simulink model "controller_stateflow"  (R2022b)
settings: Solver=FixedStepAuto  StartTime=0.0  StopTime=inf  FixedStep=0.05  RelTol=1e-3
PreLoadFcn:
  | rosinit();
model workspace (MAT data in the model file):
  SL_ROS_VariableLengthArrays_MaxSizes.CommonInfo.ArrayTruncateAction = 'EmitWarning'
  SL_ROS_VariableLengthArrays_MaxSizes.MsgTypeMap = containers.Map
  SL_ROS_VariableLengthArrays_MaxSizes.MsgTypeMap.serialization.keys = {'gazebo_msgs/LinkStates', 'trajectory_msgs/JointTrajectory', 'trajectory_msgs/JointTrajectoryPoint'}
  SL_ROS_VariableLengthArrays_MaxSizes.MsgTypeMap.serialization.values{1}(1).PropertyName = 'Name'
  SL_ROS_VariableLengthArrays_MaxSizes.MsgTypeMap.serialization.values{1}(1).DataType = 'std_msgs/String'
  SL_ROS_VariableLengthArrays_MaxSizes.MsgTypeMap.serialization.values{1}(1).MaxLength = 100
  SL_ROS_VariableLengthArrays_MaxSizes.MsgTypeMap.serialization.values{1}(2).PropertyName = 'Pose'
  SL_ROS_VariableLengthArrays_MaxSizes.MsgTypeMap.serialization.values{1}(2).DataType = 'geometry_msgs/Pose'
  SL_ROS_VariableLengthArrays_MaxSizes.MsgTypeMap.serialization.values{1}(2).MaxLength = 100
  SL_ROS_VariableLengthArrays_MaxSizes.MsgTypeMap.serialization.values{1}(3).PropertyName = 'Twist'
  SL_ROS_VariableLengthArrays_MaxSizes.MsgTypeMap.serialization.values{1}(3).DataType = 'geometry_msgs/Twist'
  SL_ROS_VariableLengthArrays_MaxSizes.MsgTypeMap.serialization.values{1}(3).MaxLength = 100
  SL_ROS_VariableLengthArrays_MaxSizes.MsgTypeMap.serialization.values{2}(1).PropertyName = 'JointNames'
  SL_ROS_VariableLengthArrays_MaxSizes.MsgTypeMap.serialization.values{2}(1).DataType = 'std_msgs/String'
  SL_ROS_VariableLengthArrays_MaxSizes.MsgTypeMap.serialization.values{2}(1).MaxLength = 16
  SL_ROS_VariableLengthArrays_MaxSizes.MsgTypeMap.serialization.values{2}(2).PropertyName = 'Points'
  SL_ROS_VariableLengthArrays_MaxSizes.MsgTypeMap.serialization.values{2}(2).DataType = 'trajectory_msgs/JointTrajectoryPoint'
  SL_ROS_VariableLengthArrays_MaxSizes.MsgTypeMap.serialization.values{2}(2).MaxLength = 5
  SL_ROS_VariableLengthArrays_MaxSizes.MsgTypeMap.serialization.values{3}(1).PropertyName = 'Accelerations'
  SL_ROS_VariableLengthArrays_MaxSizes.MsgTypeMap.serialization.values{3}(1).DataType = 'double'
  SL_ROS_VariableLengthArrays_MaxSizes.MsgTypeMap.serialization.values{3}(1).MaxLength = 128
  SL_ROS_VariableLengthArrays_MaxSizes.MsgTypeMap.serialization.values{3}(2).PropertyName = 'Effort'
  SL_ROS_VariableLengthArrays_MaxSizes.MsgTypeMap.serialization.values{3}(2).DataType = 'double'
  SL_ROS_VariableLengthArrays_MaxSizes.MsgTypeMap.serialization.values{3}(2).MaxLength = 128
  SL_ROS_VariableLengthArrays_MaxSizes.MsgTypeMap.serialization.values{3}(3).PropertyName = 'Positions'
  SL_ROS_VariableLengthArrays_MaxSizes.MsgTypeMap.serialization.values{3}(3).DataType = 'double'
  SL_ROS_VariableLengthArrays_MaxSizes.MsgTypeMap.serialization.values{3}(3).MaxLength = 7
  SL_ROS_VariableLengthArrays_MaxSizes.MsgTypeMap.serialization.values{3}(4).PropertyName = 'Velocities'
  SL_ROS_VariableLengthArrays_MaxSizes.MsgTypeMap.serialization.values{3}(4).DataType = 'double'
  SL_ROS_VariableLengthArrays_MaxSizes.MsgTypeMap.serialization.values{3}(4).MaxLength = 128
  SL_ROS_VariableLengthArrays_MaxSizes.MsgTypeMap.serialization.uniformity = 0
  SL_ROS_VariableLengthArrays_MaxSizes.MsgTypeMap.serialization.keyType = 'char'
  SL_ROS_VariableLengthArrays_MaxSizes.MsgTypeMap.serialization.valueType = 'any'
  pitch = -10
  restart = 0
undefined symbols (not defined in the file): StartTime
libraries: robotmaniplib x62, robotlib x17, robotcorelib x4, robotgazebolib x1
(part 1 of 4)
settings Model: Creator=marco  LastModifiedBy=marco
settings OptimizationCC: EnhancedBackFolding=on  PassReuseOutputArgsAs=Individual arguments  ZeroExternalMemoryAtStartup=off  ZeroInternalMemoryAtStartup=off  MaxStackSize=64  OptimizeBlockOrder=speed  DifferentSizesBufferReuse=on  OptimizationCustomize=off  EfficientTunableParamExpr=on
settings DebuggingCC: ParameterTunabilityLossMsg=error
settings HardwareCC: ProdBitPerPointer=32  ProdBitPerSizeT=32  ProdBitPerPtrDiffT=32  ProdLargestAtomicFloat=None  ProdIntDivRoundTo=Undefined  ProdEndianess=Unspecified  ProdWordSize=32  ProdHWDeviceType=Generic->Unspecified (assume 32-bit Generic)
settings SFSimCC: MATLABDynamicMemAlloc=off
settings RTWCC: Description=Embedded Coder  SystemTargetFile=ert.tlc  HardwareBoard=Robot Operating System (ROS)  TLCOptions="-aInlineSetEventsForThisBaseRateFcn=TLC_FALSE -aSuppressMultiTaskScheduler=TLC_FALSE  -aRateBasedStepFcn=0"  TemplateMakefile=ert_default_tmf  Toolchain=Catkin  TargetLang=C++
settings CodeAppCC: ForceParamTrailComments=on  IgnoreCustomStorageClasses=off  OperatorAnnotations=on  SimulinkDataObjDesc=on  SFDataObjDesc=on  InsertBlockDesc=on

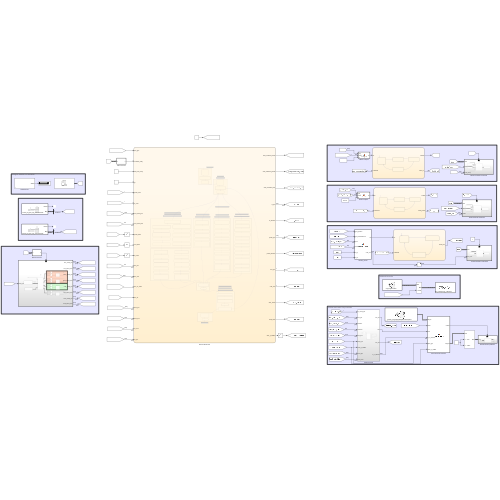
[thumbnail: Simulink's stored preview of the top-level diagram]
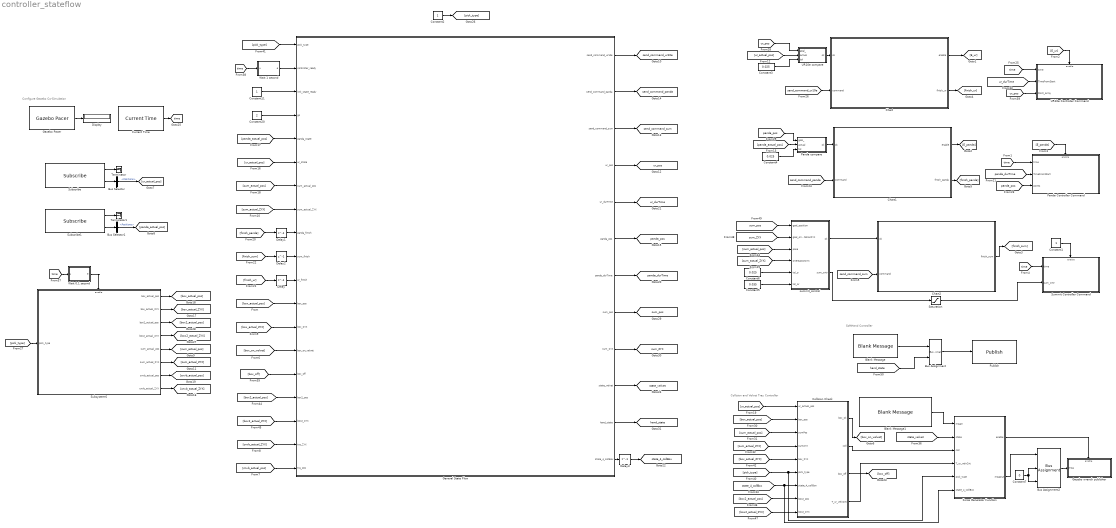
== system controller_stateflow ==
  note: Collision and Velvet Tray Controller
  note: SoftHand Controller
  note: Configure Gazebo Co-Simulation
  Blank Message : robotlib/Blank Message  messageClass=Message  entityType=std_msgs/Float64  messageType=std_msgs/Float64  SampleTime=inf  legacyBusStruct=off
      settings: LibrarySourceBlock=roslib/ROS/Blank Message
  Blank Message1 : robotlib/Blank Message  messageClass=Service Request  entityType=gazebo_msgs/ApplyBodyWrench  messageType=gazebo_msgs/ApplyBodyWrenchRequest  SampleTime=-1  legacyBusStruct=off
      settings: LibrarySourceBlock=roslib/ROS/Blank Message
  Bus Assignment : BusAssignment  AssignedSignals=Data
  Bus Assignment2 : BusAssignment  AssignedSignals=StartTime.Sec,StartTime.Nsec
  Bus Selector : BusSelector  OutputSignals=Actual.Positions
  Bus Selector1 : BusSelector  OutputSignals=Actual.Positions
  Chart : Stateflow chart  TreatAsAtomicUnit=on
  Chart1 : Stateflow chart  TreatAsAtomicUnit=on
  Chart2 : Stateflow chart  TreatAsAtomicUnit=on
  Collision Check : Subsystem
  Constant1 : Constant
  Constant11 : Constant
  Constant2 : Constant
  Constant20 : Constant  Value=2
  Constant3 : Constant  Value=0.025
  Constant4 : Constant  Value=0.025
  Constant5 : Constant  Value=0.035
  Constant6 : Constant  Value=0.025
  Constant7 : Constant  Value=0
  Current Time : robotlib/Current Time  OutputFormat=bus  SampleTime=-1  ModelName=controller_stateflow
      settings: LibrarySourceBlock=roslib/ROS/Current Time
  Delay{,1..3} (4 alike) : Delay  DelayLength=1  InitialCondition=0
  Display : Display
  Force Generator Function : MATLAB Function  TreatAsAtomicUnit=on
  Gazebo Pacer : robotgazebolib/Gazebo Pacer  ResetBehavior=Reset Gazebo simulation time  SampleTime=0.05
  Gazebo wrench publisher : Subsystem
  General State Flow : Stateflow chart  TreatAsAtomicUnit=on
  Panda Controller Command : Subsystem
  Panda compare : MATLAB Function  TreatAsAtomicUnit=on
  Publish : robotlib/Publish  topicSource=Select from ROS network  topic=/right_hand_v1s/synergy_command  messageType=std_msgs/Float64  legacyBusStruct=off  messageQueueLength=1
      settings: LibrarySourceBlock=roslib/ROS/Publish
  Saturation : Saturate  UpperLimit=0.3  LowerLimit=-0.3
  Subscribe : robotlib/Subscribe  topicSource=Select from ROS network  topic=/ur10e_eff_joint_traj_controller/state  messageType=control_msgs/JointTrajectoryControllerState  SampleTime=-1  legacyBusStruct=off  messageQueueLength=1
      settings: LibrarySourceBlock=roslib/ROS/Subscribe
  Subscribe1 : robotlib/Subscribe  topicSource=Select from ROS network  topic=/panda_eff_joint_traj_controller/state  messageType=control_msgs/JointTrajectoryControllerState  SampleTime=-1  legacyBusStruct=off  messageQueueLength=1
      settings: LibrarySourceBlock=roslib/ROS/Subscribe
  Subsystem6 : Subsystem
  Summit Controller Command : Subsystem
  Terminator : Terminator
  Terminator1 : Terminator
  UR10e Controller Command : Subsystem
  UR10e compare : MATLAB Function  TreatAsAtomicUnit=on
  Wait 0,1 second : MATLAB Function  TreatAsAtomicUnit=on
  Wait 1 second : MATLAB Function  TreatAsAtomicUnit=on
  summit_control : MATLAB Function  TreatAsAtomicUnit=on
  tag scope: hand_state=global, panda_durTime=global, panda_pos=global, send_command_panda=global, send_command_sum=global, send_command_ur10e=global, state_4_collBox=global, state_velvet=global, sum_ZYX=global, sum_pos=global, time=global, ur_durTime=global, ur_pos=global
  wires:
  [time] -> Panda Controller Command/1(time)
  [E_ur] -> UR10e Controller Command/Enable
  Chart/1(enable) -> [E_ur]
  Subscribe/2 -> Bus Selector/1
  Constant3/1 -> UR10e compare/3(tol)
  UR10e compare/1(ok) -> Chart/1(ok)
  Panda compare/1(ok) -> Chart1/1(ok)
  Constant4/1 -> Panda compare/3(tol)
  Subscribe1/2 -> Bus Selector1/1
  [panda_pos] -> Panda Controller Command/3(points)
  Constant6/1 -> summit_control/5(tol_p)
  summit_control/1(ok) -> Chart2/1(ok)
  summit_control/2(sum_cntr) -> Saturation/1
  Constant1/1 -> Summit Controller Command/Enable
  Chart/2(finish_ur) -> [finish_ur]
  Saturation/1 -> Summit Controller Command/2(sum_cntr)
  Wait 0,1 second/1(e) -> Subsystem6/Enable
  Constant11/1 -> General State Flow/3(link_state_ready)
  Bus Selector/1 -> [ur_actual_pos]  "<Positions>"
  Bus Selector1/1 -> [panda_actual_pos]  "<Positions>"
  [ur_actual_pos] -> UR10e compare/2(actual)
  [sum_actual_ZYX] -> summit_control/4(orientationZYX)
  [panda_actual_pos] -> Panda compare/2(actual)
  [panda_actual_pos] -> General State Flow/5(panda_state)
  [ur_actual_pos] -> General State Flow/6(ur_state)
  [finish_sum] -> Delay2/1
  [finish_ur] -> Delay/1
  Delay/1 -> General State Flow/11(ur_finish)
  Constant20/1 -> General State Flow/4(go)
  [time] -> UR10e Controller Command/1(time)
  General State Flow/1(send_command_ur10e) -> [send_command_ur10e]
  [send_command_ur10e] -> Chart/2(command)
  [ur_pos] -> UR10e compare/1(goal_)
  General State Flow/3(send_command_sum) -> [send_command_sum]
  General State Flow/2(send_command_panda) -> [send_command_panda]
  General State Flow/4(ur_pos) -> [ur_pos]
  General State Flow/6(panda_pos) -> [panda_pos]
  [send_command_panda] -> Chart1/2(command)
  [panda_pos] -> Panda compare/1(goal_)
  [finish_panda] -> Delay1/1
  Delay1/1 -> General State Flow/9(panda_finish)
  [time] -> Summit Controller Command/1(time)
  [send_command_sum] -> Chart2/2(command)
  Chart2/1(finish_sum) -> [finish_sum]
  Delay2/1 -> General State Flow/10(sum_finish)
  [box_actual_ZYX] -> General State Flow/13(box_ZYX)
  [box_actual_pos] -> General State Flow/12(box_pos)
  [sum_actual_pos] -> summit_control/3(pose)
  [sum_actual_ZYX] -> General State Flow/8(sum_actual_ZYX)
  [sum_actual_pos] -> General State Flow/7(sum_actual_pos)
  [box_on_velvet] -> General State Flow/14(box_on_velvet)
  Bus Assignment/1 -> Publish/1
  Blank Message/1 -> Bus Assignment/1
  [cnvb_actual_pos] -> General State Flow/19(tra_pos)
  [cnvb_actual_ZYX] -> General State Flow/18(tra_ZYX)
  [E_panda] -> Panda Controller Command/Enable
  [panda_durTime] -> Panda Controller Command/2(TimeFromStart)
  General State Flow/5(ur_durTime) -> [ur_durTime]
  [ur_durTime] -> UR10e Controller Command/2(TimeFromStart)
  General State Flow/7(panda_durTime) -> [panda_durTime]
  Force Generator Function/1(enable) -> Gazebo wrench publisher/Enable
  Blank Message1/1 -> Force Generator Function/1(msgIn)
  Bus Assignment2/1 -> Gazebo wrench publisher/1(msg)
  Constant7/1 -> Bus Assignment2/3, Bus Assignment2/2
  Force Generator Function/2(msgOut) -> Bus Assignment2/1
  [box_off] -> General State Flow/15(box_off)
  General State Flow/10(state_velvet) -> [state_velvet]
  [ur_actual_pos] -> Collision Check/1(ur_actual_pos)
  [box_actual_pos] -> Collision Check/2(box_pos)
  [sum_actual_pos] -> Collision Check/3(sumPos)
  [sum_actual_ZYX] -> Collision Check/4(sumZYX)
  Collision Check/1(box_ok) -> [box_on_velvet]
  Collision Check/2(coll) -> Force Generator Function/3(coll)
  Collision Check/3(box_off) -> [box_off]
  Collision Check/4(T_ur_velvCnt) -> Force Generator Function/4(T_ur_velvCnt)
  Gazebo Pacer/1 -> Display/1
  Subsystem6/5(sum_actual_pos) -> [sum_actual_pos]
  Subsystem6/6(sum_actual_ZYX) -> [sum_actual_ZYX]
  Subsystem6/7(cnvb_actual_pos) -> [cnvb_actual_pos]
  Subsystem6/8(cnvb_actual_ZYX) -> [cnvb_actual_ZYX]
  [time] -> Wait 0,1 second/1(u)
  Current Time/1 -> [time]
  [time] -> Wait 1 second/1(u)
  Wait 1 second/1(e) -> General State Flow/2(controller_ready)
  [ur_pos] -> UR10e Controller Command/3(Point_array)
  Constant2/1 -> [pick_type]
  Subsystem6/1(box_actual_pos) -> [box_actual_pos]
  Subsystem6/2(box_actual_ZYX) -> [box_actual_ZYX]
  [pick_type] -> Subsystem6/1(pick_type)
  [pick_type] -> Collision Check/6(pick_type), Force Generator Function/5(pick_type)
  [pick_type] -> General State Flow/1(pick_type)
  [box_actual_ZYX] -> Collision Check/5(box_ZYX)
  [state_velvet] -> Force Generator Function/2(state)
  Subsystem6/3(box2_actual_pos) -> [box2_actual_pos]
  Subsystem6/4(box2_actual_ZYX) -> [box2_actual_ZYX]
  [box2_actual_ZYX] -> General State Flow/17(box2_ZYX)
  [box2_actual_pos] -> General State Flow/16(box2_pos)
  [box2_actual_pos] -> Collision Check/8(box2_pos)
  [box2_actual_ZYX] -> Collision Check/9(box2_ZYX)
  General State Flow/12(state_4_collBox) -> Delay3/1
  Subscribe/1 -> Terminator/1
  Subscribe1/1 -> Terminator1/1
  General State Flow/9(sum_ZYX) -> [sum_ZYX]
  [sum_ZYX] -> summit_control/2(goal_orientationZYX)
  General State Flow/8(sum_pos) -> [sum_pos]
  [sum_pos] -> summit_control/1(goal_position)
  Constant5/1 -> summit_control/6(tol_or)
  General State Flow/11(hand_state) -> [hand_state]
  [hand_state] -> Bus Assignment/2
  Chart1/2(finish_panda) -> [finish_panda]
  Chart1/1(enable) -> [E_panda]
  Delay3/1 -> [state_4_collBox]
  [state_4_collBox] -> Collision Check/7(state_4_collBox), Force Generator Function/6(state_4_collBox)

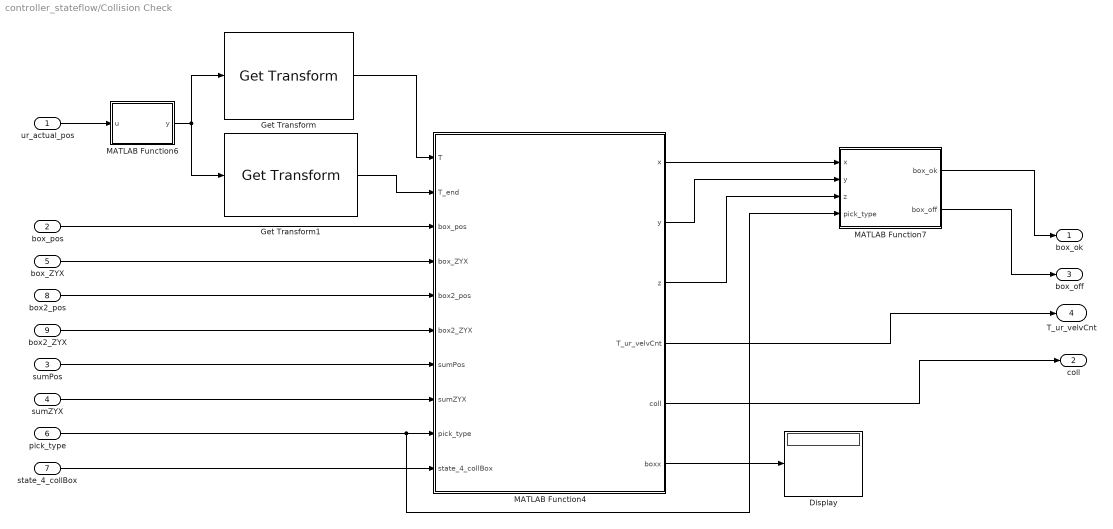
== system controller_stateflow/Collision Check ==
  ur_actual_pos : Inport
  box_pos : Inport  Port=2
  sumPos : Inport  Port=3
  sumZYX : Inport  Port=4
  box_ZYX : Inport  Port=5  OutDataTypeStr=double  PortDimensions=[3,1]
  pick_type : Inport  Port=6
  state_4_collBox : Inport  Port=7
  box2_pos : Inport  Port=8
  box2_ZYX : Inport  Port=9  OutDataTypeStr=double  PortDimensions=[3,1]
  Display : Display
  Get Transform : robotmaniplib/Get Transform  RigidBodyTree=ur10e  SourceBody=ee_link  TargetBody=world  SimulateUsing=Interpreted execution
  Get Transform1 : robotmaniplib/Get Transform  RigidBodyTree=ur10e  SourceBody=velvet_link_end  TargetBody=world  SimulateUsing=Interpreted execution
  MATLAB Function4 : MATLAB Function  TreatAsAtomicUnit=on
  MATLAB Function6 : MATLAB Function  TreatAsAtomicUnit=on
  MATLAB Function7 : MATLAB Function  TreatAsAtomicUnit=on
  box_ok : Outport
  coll : Outport  Port=2
  box_off : Outport  Port=3
  T_ur_velvCnt : Outport  Port=4
  wires:
  MATLAB Function7/1(box_ok) -> box_ok/1
  Get Transform/1 -> MATLAB Function4/1(T)
  MATLAB Function4/1(x) -> MATLAB Function7/1(x)
  MATLAB Function7/2(box_off) -> box_off/1
  MATLAB Function4/3(z) -> MATLAB Function7/3(z)
  MATLAB Function4/2(y) -> MATLAB Function7/2(y)
  MATLAB Function4/5(coll) -> coll/1
  box_pos/1 -> MATLAB Function4/3(box_pos)
  ur_actual_pos/1 -> MATLAB Function6/1(u)
  sumPos/1 -> MATLAB Function4/7(sumPos)
  MATLAB Function4/4(T_ur_velvCnt) -> T_ur_velvCnt/1
  sumZYX/1 -> MATLAB Function4/8(sumZYX)
  MATLAB Function4/6(boxx) -> Display/1
  pick_type/1 -> MATLAB Function7/4(pick_type), MATLAB Function4/9(pick_type)
  MATLAB Function6/1(y) -> Get Transform/1, Get Transform1/1
  box_ZYX/1 -> MATLAB Function4/4(box_ZYX)
  Get Transform1/1 -> MATLAB Function4/2(T_end)
  box2_ZYX/1 -> MATLAB Function4/6(box2_ZYX)
  box2_pos/1 -> MATLAB Function4/5(box2_pos)
  state_4_collBox/1 -> MATLAB Function4/10(state_4_collBox)

== system controller_stateflow/Gazebo wrench publisher ==
  msg : Inport
  Enable : EnablePort
  Call Service : robotlib/Call Service  topicSource=Select from ROS network  service=/gazebo/apply_body_wrench  serviceType=gazebo_msgs/ApplyBodyWrench  connectionTimeout=5  keepPersistent=off  ShowErrorCodeOutput=on  legacyBusStruct=off
      settings: LibrarySourceBlock=roslib/ROS/Call Service
  Terminator : Terminator
  Terminator1 : Terminator
  wires:
  Call Service/1 -> Terminator/1
  Call Service/2 -> Terminator1/1
  msg/1 -> Call Service/1

== system controller_stateflow/General State Flow/THE_END ==
  go : Inport
  Action Port : ActionPort
      settings: CopyFcn=Stateflow.SLINSF.SimulinkMan.removeBlockPreDeleteFcn  PreDeleteFcn=Stateflow.SLINSF.SimulinkMan.unsafePredeleteFcn
  Stop Simulation : Stop
  wires:
  go/1 -> Stop Simulation/1

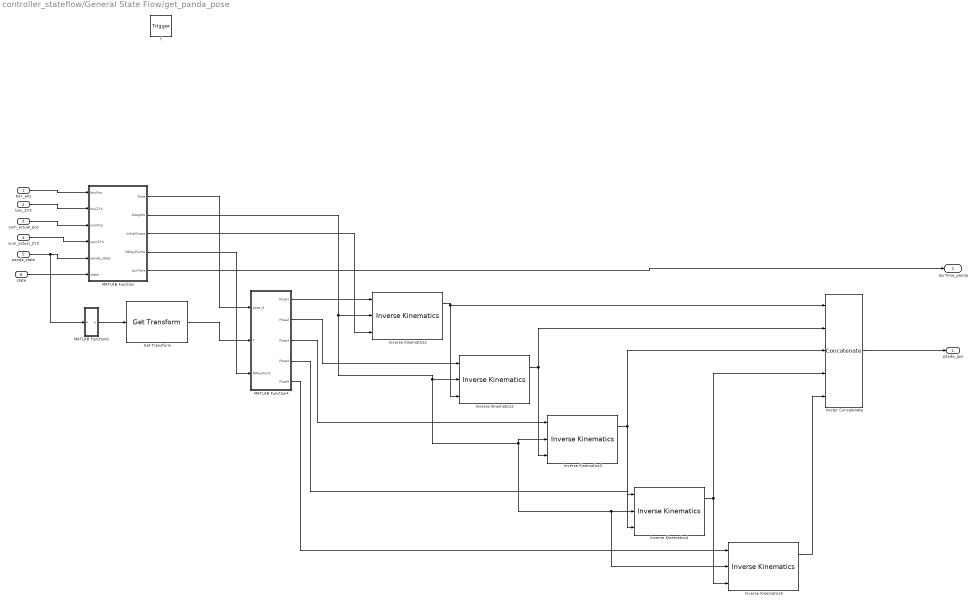
== system controller_stateflow/General State Flow/get_panda_pose ==
  box_pos : Inport  OutDataTypeStr=double  PortDimensions=[3,1]
  box_ZYX : Inport  Port=2  OutDataTypeStr=double  PortDimensions=[3,1]
  sum_actual_pos : Inport  Port=3  OutDataTypeStr=double  PortDimensions=[3,1]
  sum_actual_ZYX : Inport  Port=4  OutDataTypeStr=double  PortDimensions=[3,1]
  panda_state : Inport  Port=5  OutDataTypeStr=double  PortDimensions=[7,1]
  state : Inport  Port=6  OutDataTypeStr=double  PortDimensions=1
  f : TriggerPort  TriggerType=function-call  VariantControl=(inherit)
      settings: CopyFcn=Stateflow.SLINSF.SimulinkMan.removeBlockPreDeleteFcn  PreDeleteFcn=Stateflow.SLINSF.SimulinkMan.unsafePredeleteFcn
  Get Transform : robotmaniplib/Get Transform  RigidBodyTree=franka  SourceBody=hand_link_end  TargetBody=panda_link0  SimulateUsing=Interpreted execution
  Inverse Kinematics{1..5} (5 alike) : robotmaniplib/Inverse Kinematics  RigidBodyTree=franka  EndEffector=hand_link_end  ShowInfo=on  SolverName=BFGS Gradient Projection  EnforceJointLimits=on  MaxIterations=1500  MaxTime=10  GradientTolerance=1e-7  SolutionTolerance=1e-6  StepTolerance=1e-14  ErrorChangeTolerance=1e-12  UseErrorDamping=on  DampingBias=0.0025  SimulateUsing=Interpreted execution
  MATLAB Function : MATLAB Function  TreatAsAtomicUnit=on
  MATLAB Function4 : MATLAB Function  TreatAsAtomicUnit=on
  MATLAB Function6 : MATLAB Function  TreatAsAtomicUnit=on
  Vector Concatenate : Concatenate  NumInputs=5  Mode=Multidimensional array  ConcatenateDimension=2
  panda_pos : Outport
  durTime_panda : Outport  Port=2
  wires:
  panda_state/1 -> MATLAB Function6/1(u), MATLAB Function/5(panda_state)
  box_pos/1 -> MATLAB Function/1(boxPos)
  box_ZYX/1 -> MATLAB Function/2(boxZYX)
  sum_actual_pos/1 -> MATLAB Function/3(sumPos)
  sum_actual_ZYX/1 -> MATLAB Function/4(sumZYX)
  state/1 -> MATLAB Function/6(state)
  MATLAB Function/5(durTime) -> durTime_panda/1
  MATLAB Function/4(NWayPoints) -> MATLAB Function4/3(NWayPoint)
  Inverse Kinematics3/1 -> Inverse Kinematics4/3, Vector Concatenate/3
  MATLAB Function6/1(y) -> Get Transform/1
  Vector Concatenate/1 -> panda_pos/1
  MATLAB Function4/1(Pose1) -> Inverse Kinematics1/1
  MATLAB Function4/2(Pose2) -> Inverse Kinematics2/1
  MATLAB Function/3(initialGuess) -> Inverse Kinematics1/3
  MATLAB Function/2(Weights) -> Inverse Kinematics2/2, Inverse Kinematics3/2, Inverse Kinematics5/2, Inverse Kinematics4/2, Inverse Kinematics1/2
  MATLAB Function/1(Pose) -> MATLAB Function4/1(pose_d)
  MATLAB Function4/3(Pose3) -> Inverse Kinematics3/1
  Inverse Kinematics1/1 -> Inverse Kinematics2/3, Vector Concatenate/1
  Get Transform/1 -> MATLAB Function4/2(T)
  Inverse Kinematics2/1 -> Inverse Kinematics3/3, Vector Concatenate/2
  Inverse Kinematics4/1 -> Inverse Kinematics5/3, Vector Concatenate/4
  Inverse Kinematics5/1 -> Vector Concatenate/5
  MATLAB Function4/4(Pose4) -> Inverse Kinematics4/1
  MATLAB Function4/5(Pose5) -> Inverse Kinematics5/1

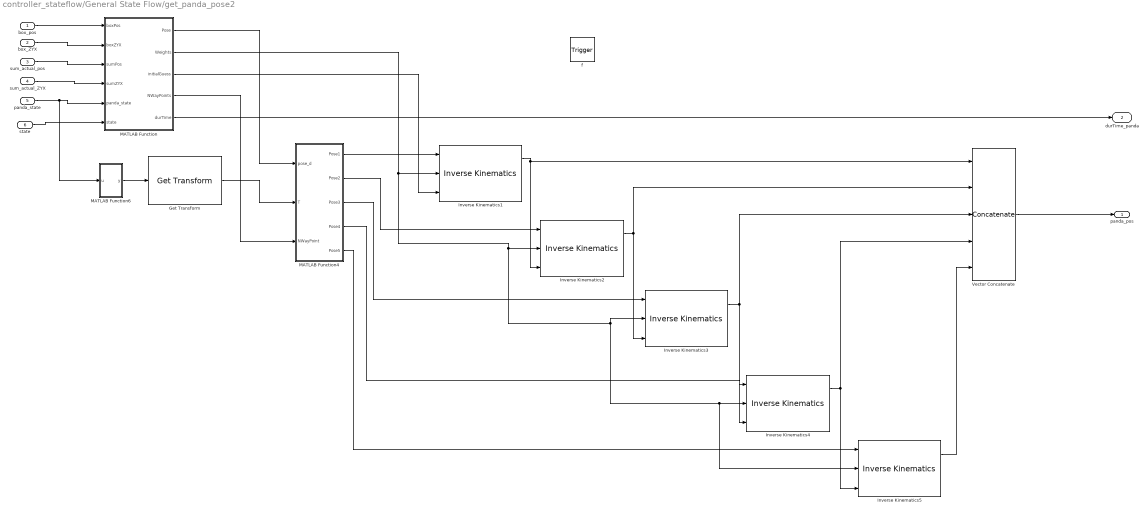
== system controller_stateflow/General State Flow/get_panda_pose2 ==
  box_pos : Inport  OutDataTypeStr=double  PortDimensions=[3,1]
  box_ZYX : Inport  Port=2  OutDataTypeStr=double  PortDimensions=[3,1]
  sum_actual_pos : Inport  Port=3  OutDataTypeStr=double  PortDimensions=[3,1]
  sum_actual_ZYX : Inport  Port=4  OutDataTypeStr=double  PortDimensions=[3,1]
  panda_state : Inport  Port=5  OutDataTypeStr=double  PortDimensions=[7,1]
  state : Inport  Port=6  OutDataTypeStr=double  PortDimensions=1
  f : TriggerPort  TriggerType=function-call  VariantControl=(inherit)
      settings: CopyFcn=Stateflow.SLINSF.SimulinkMan.removeBlockPreDeleteFcn  PreDeleteFcn=Stateflow.SLINSF.SimulinkMan.unsafePredeleteFcn
  Get Transform : robotmaniplib/Get Transform  RigidBodyTree=franka  SourceBody=hand_link_end  TargetBody=panda_link0  SimulateUsing=Interpreted execution
  Inverse Kinematics{1..5} (5 alike) : robotmaniplib/Inverse Kinematics  RigidBodyTree=franka  EndEffector=hand_link_end  ShowInfo=on  SolverName=BFGS Gradient Projection  EnforceJointLimits=on  MaxIterations=1500  MaxTime=10  GradientTolerance=1e-7  SolutionTolerance=1e-6  StepTolerance=1e-14  ErrorChangeTolerance=1e-12  UseErrorDamping=on  DampingBias=0.0025  SimulateUsing=Interpreted execution
  MATLAB Function : MATLAB Function  TreatAsAtomicUnit=on
  MATLAB Function4 : MATLAB Function  TreatAsAtomicUnit=on
  MATLAB Function6 : MATLAB Function  TreatAsAtomicUnit=on
  Vector Concatenate : Concatenate  NumInputs=5  Mode=Multidimensional array  ConcatenateDimension=2
  panda_pos : Outport
  durTime_panda : Outport  Port=2
  wires:
  panda_state/1 -> MATLAB Function6/1(u), MATLAB Function/5(panda_state)
  box_pos/1 -> MATLAB Function/1(boxPos)
  box_ZYX/1 -> MATLAB Function/2(boxZYX)
  sum_actual_pos/1 -> MATLAB Function/3(sumPos)
  sum_actual_ZYX/1 -> MATLAB Function/4(sumZYX)
  state/1 -> MATLAB Function/6(state)
  MATLAB Function/5(durTime) -> durTime_panda/1
  MATLAB Function/4(NWayPoints) -> MATLAB Function4/3(NWayPoint)
  Inverse Kinematics3/1 -> Inverse Kinematics4/3, Vector Concatenate/3
  MATLAB Function6/1(y) -> Get Transform/1
  Vector Concatenate/1 -> panda_pos/1
  MATLAB Function4/1(Pose1) -> Inverse Kinematics1/1
  MATLAB Function4/2(Pose2) -> Inverse Kinematics2/1
  MATLAB Function/3(initialGuess) -> Inverse Kinematics1/3
  MATLAB Function/2(Weights) -> Inverse Kinematics2/2, Inverse Kinematics3/2, Inverse Kinematics5/2, Inverse Kinematics4/2, Inverse Kinematics1/2
  MATLAB Function/1(Pose) -> MATLAB Function4/1(pose_d)
  MATLAB Function4/3(Pose3) -> Inverse Kinematics3/1
  Inverse Kinematics1/1 -> Inverse Kinematics2/3, Vector Concatenate/1
  Get Transform/1 -> MATLAB Function4/2(T)
  Inverse Kinematics2/1 -> Inverse Kinematics3/3, Vector Concatenate/2
  Inverse Kinematics4/1 -> Inverse Kinematics5/3, Vector Concatenate/4
  Inverse Kinematics5/1 -> Vector Concatenate/5
  MATLAB Function4/4(Pose4) -> Inverse Kinematics4/1
  MATLAB Function4/5(Pose5) -> Inverse Kinematics5/1

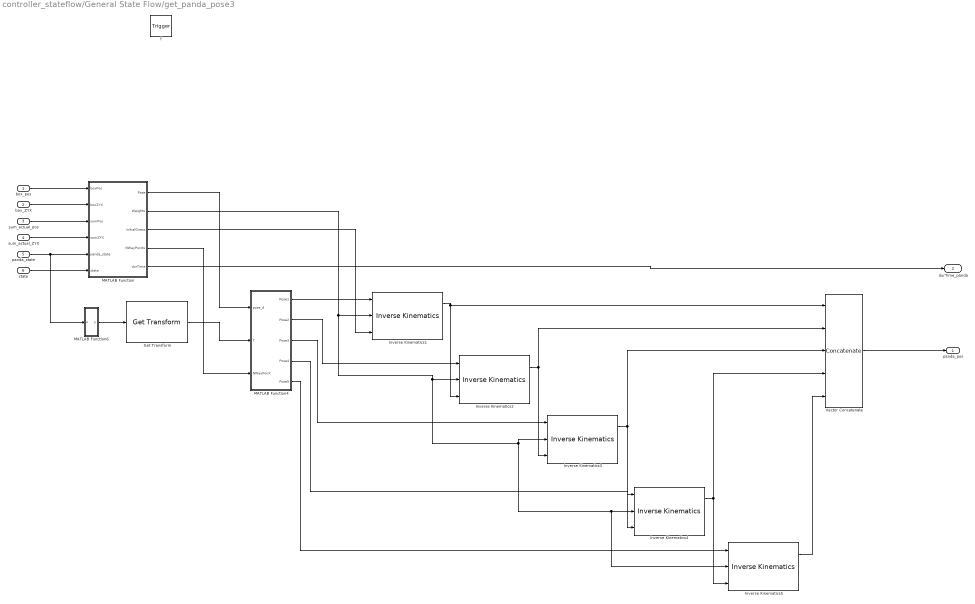
== system controller_stateflow/General State Flow/get_panda_pose3 ==
  box_pos : Inport  OutDataTypeStr=double  PortDimensions=[3,1]
  box_ZYX : Inport  Port=2  OutDataTypeStr=double  PortDimensions=[3,1]
  sum_actual_pos : Inport  Port=3  OutDataTypeStr=double  PortDimensions=[3,1]
  sum_actual_ZYX : Inport  Port=4  OutDataTypeStr=double  PortDimensions=[3,1]
  panda_state : Inport  Port=5  OutDataTypeStr=double  PortDimensions=[7,1]
  state : Inport  Port=6  OutDataTypeStr=double  PortDimensions=1
  f : TriggerPort  TriggerType=function-call  VariantControl=(inherit)
      settings: CopyFcn=Stateflow.SLINSF.SimulinkMan.removeBlockPreDeleteFcn  PreDeleteFcn=Stateflow.SLINSF.SimulinkMan.unsafePredeleteFcn
  Get Transform : robotmaniplib/Get Transform  RigidBodyTree=franka  SourceBody=hand_link_end  TargetBody=panda_link0  SimulateUsing=Interpreted execution
  Inverse Kinematics{1..5} (5 alike) : robotmaniplib/Inverse Kinematics  RigidBodyTree=franka  EndEffector=hand_link_end  ShowInfo=on  SolverName=BFGS Gradient Projection  EnforceJointLimits=on  MaxIterations=1500  MaxTime=10  GradientTolerance=1e-7  SolutionTolerance=1e-6  StepTolerance=1e-14  ErrorChangeTolerance=1e-12  UseErrorDamping=on  DampingBias=0.0025  SimulateUsing=Interpreted execution
  MATLAB Function : MATLAB Function  TreatAsAtomicUnit=on
  MATLAB Function4 : MATLAB Function  TreatAsAtomicUnit=on
  MATLAB Function6 : MATLAB Function  TreatAsAtomicUnit=on
  Vector Concatenate : Concatenate  NumInputs=5  Mode=Multidimensional array  ConcatenateDimension=2
  panda_pos : Outport
  durTime_panda : Outport  Port=2
  wires:
  panda_state/1 -> MATLAB Function6/1(u), MATLAB Function/5(panda_state)
  box_pos/1 -> MATLAB Function/1(boxPos)
  box_ZYX/1 -> MATLAB Function/2(boxZYX)
  sum_actual_pos/1 -> MATLAB Function/3(sumPos)
  sum_actual_ZYX/1 -> MATLAB Function/4(sumZYX)
  state/1 -> MATLAB Function/6(state)
  MATLAB Function/5(durTime) -> durTime_panda/1
  MATLAB Function/4(NWayPoints) -> MATLAB Function4/3(NWayPoint)
  Inverse Kinematics3/1 -> Inverse Kinematics4/3, Vector Concatenate/3
  MATLAB Function6/1(y) -> Get Transform/1
  Vector Concatenate/1 -> panda_pos/1
  MATLAB Function4/1(Pose1) -> Inverse Kinematics1/1
  MATLAB Function4/2(Pose2) -> Inverse Kinematics2/1
  MATLAB Function/3(initialGuess) -> Inverse Kinematics1/3
  MATLAB Function/2(Weights) -> Inverse Kinematics2/2, Inverse Kinematics3/2, Inverse Kinematics5/2, Inverse Kinematics4/2, Inverse Kinematics1/2
  MATLAB Function/1(Pose) -> MATLAB Function4/1(pose_d)
  MATLAB Function4/3(Pose3) -> Inverse Kinematics3/1
  Inverse Kinematics1/1 -> Inverse Kinematics2/3, Vector Concatenate/1
  Get Transform/1 -> MATLAB Function4/2(T)
  Inverse Kinematics2/1 -> Inverse Kinematics3/3, Vector Concatenate/2
  Inverse Kinematics4/1 -> Inverse Kinematics5/3, Vector Concatenate/4
  Inverse Kinematics5/1 -> Vector Concatenate/5
  MATLAB Function4/4(Pose4) -> Inverse Kinematics4/1
  MATLAB Function4/5(Pose5) -> Inverse Kinematics5/1

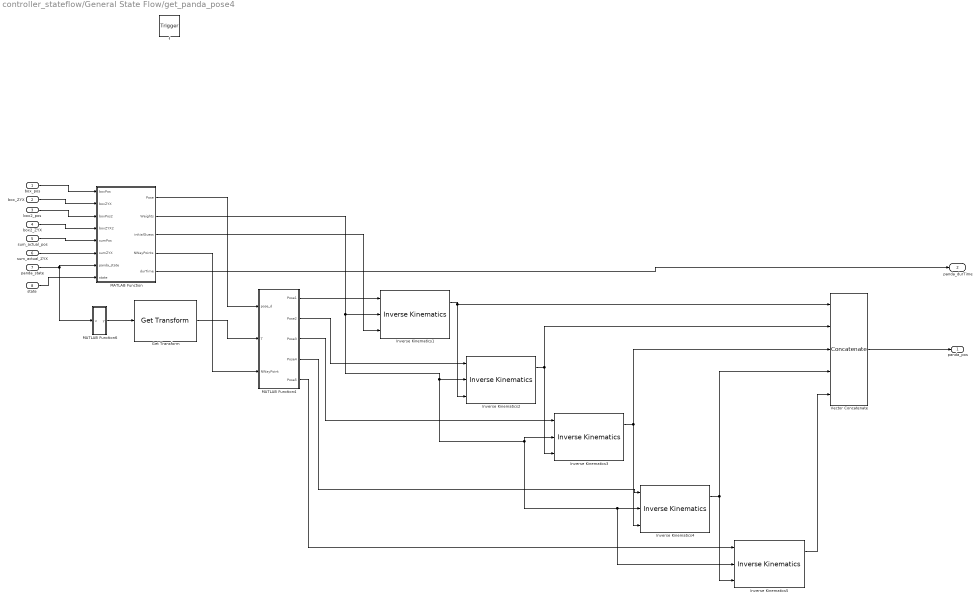
== system controller_stateflow/General State Flow/get_panda_pose4 ==
  box_pos : Inport  OutDataTypeStr=double  PortDimensions=[3,1]
  box_ZYX : Inport  Port=2  OutDataTypeStr=double  PortDimensions=[3,1]
  box2_pos : Inport  Port=3  OutDataTypeStr=double  PortDimensions=[3,1]
  box2_ZYX : Inport  Port=4  OutDataTypeStr=double  PortDimensions=[3,1]
  sum_actual_pos : Inport  Port=5  OutDataTypeStr=double  PortDimensions=[3,1]
  sum_actual_ZYX : Inport  Port=6  OutDataTypeStr=double  PortDimensions=[3,1]
  panda_state : Inport  Port=7  OutDataTypeStr=double  PortDimensions=[7,1]
  state : Inport  Port=8  OutDataTypeStr=double  PortDimensions=1
  f : TriggerPort  TriggerType=function-call  VariantControl=(inherit)
      settings: CopyFcn=Stateflow.SLINSF.SimulinkMan.removeBlockPreDeleteFcn  PreDeleteFcn=Stateflow.SLINSF.SimulinkMan.unsafePredeleteFcn
  Get Transform : robotmaniplib/Get Transform  RigidBodyTree=franka  SourceBody=hand_link_end  TargetBody=panda_link0  SimulateUsing=Interpreted execution
  Inverse Kinematics{1..5} (5 alike) : robotmaniplib/Inverse Kinematics  RigidBodyTree=franka  EndEffector=hand_link_end  ShowInfo=on  SolverName=BFGS Gradient Projection  EnforceJointLimits=on  MaxIterations=1500  MaxTime=10  GradientTolerance=1e-7  SolutionTolerance=1e-6  StepTolerance=1e-14  ErrorChangeTolerance=1e-12  UseErrorDamping=on  DampingBias=0.0025  SimulateUsing=Interpreted execution
  MATLAB Function : MATLAB Function  TreatAsAtomicUnit=on
  MATLAB Function4 : MATLAB Function  TreatAsAtomicUnit=on
  MATLAB Function6 : MATLAB Function  TreatAsAtomicUnit=on
  Vector Concatenate : Concatenate  NumInputs=5  Mode=Multidimensional array  ConcatenateDimension=2
  panda_pos : Outport
  panda_durTime : Outport  Port=2
  wires:
  panda_state/1 -> MATLAB Function/7(panda_state), MATLAB Function6/1(u)
  box_pos/1 -> MATLAB Function/1(boxPos)
  box_ZYX/1 -> MATLAB Function/2(boxZYX)
  sum_actual_pos/1 -> MATLAB Function/5(sumPos)
  sum_actual_ZYX/1 -> MATLAB Function/6(sumZYX)
  state/1 -> MATLAB Function/8(state)
  MATLAB Function/5(durTime) -> panda_durTime/1
  MATLAB Function/4(NWayPoints) -> MATLAB Function4/3(NWayPoint)
  Inverse Kinematics3/1 -> Inverse Kinematics4/3, Vector Concatenate/3
  MATLAB Function6/1(y) -> Get Transform/1
  Vector Concatenate/1 -> panda_pos/1
  MATLAB Function4/1(Pose1) -> Inverse Kinematics1/1
  MATLAB Function4/2(Pose2) -> Inverse Kinematics2/1
  MATLAB Function/3(initialGuess) -> Inverse Kinematics1/3
  MATLAB Function/2(Weights) -> Inverse Kinematics2/2, Inverse Kinematics3/2, Inverse Kinematics5/2, Inverse Kinematics4/2, Inverse Kinematics1/2
  MATLAB Function/1(Pose) -> MATLAB Function4/1(pose_d)
  MATLAB Function4/3(Pose3) -> Inverse Kinematics3/1
  Inverse Kinematics1/1 -> Inverse Kinematics2/3, Vector Concatenate/1
  Get Transform/1 -> MATLAB Function4/2(T)
  Inverse Kinematics2/1 -> Vector Concatenate/2, Inverse Kinematics3/3
  Inverse Kinematics4/1 -> Inverse Kinematics5/3, Vector Concatenate/4
  Inverse Kinematics5/1 -> Vector Concatenate/5
  MATLAB Function4/4(Pose4) -> Inverse Kinematics4/1
  MATLAB Function4/5(Pose5) -> Inverse Kinematics5/1
  box2_pos/1 -> MATLAB Function/3(boxPos2)
  box2_ZYX/1 -> MATLAB Function/4(boxZYX2)

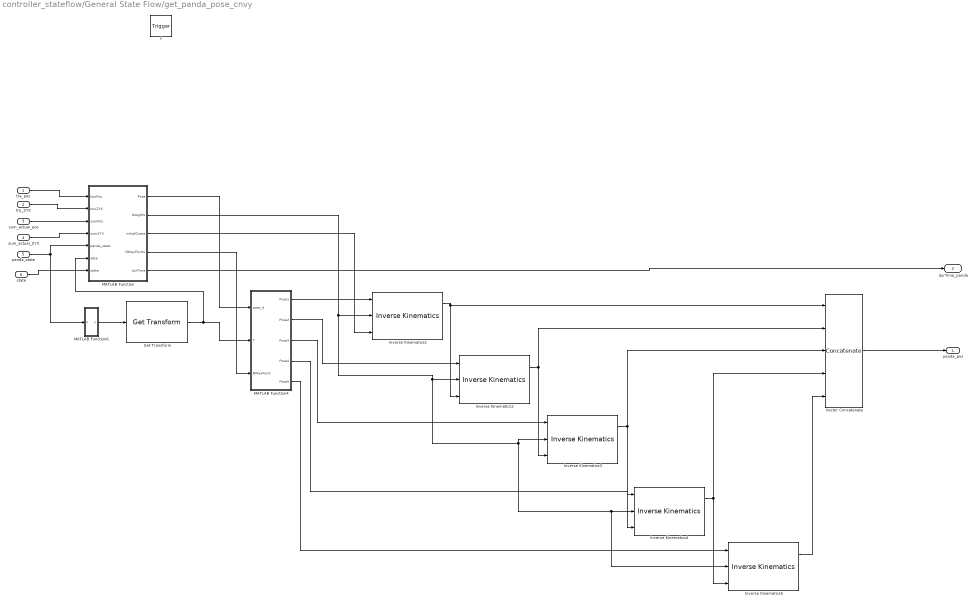
== system controller_stateflow/General State Flow/get_panda_pose_cnvy ==
  tra_pos : Inport  OutDataTypeStr=double  PortDimensions=[3,1]
  tra_ZYX : Inport  Port=2  OutDataTypeStr=double  PortDimensions=[3,1]
  sum_actual_pos : Inport  Port=3  OutDataTypeStr=double  PortDimensions=[3,1]
  sum_actual_ZYX : Inport  Port=4  OutDataTypeStr=double  PortDimensions=[3,1]
  panda_state : Inport  Port=5  OutDataTypeStr=double  PortDimensions=[7,1]
  state : Inport  Port=6  OutDataTypeStr=double  PortDimensions=1
  f : TriggerPort  TriggerType=function-call  VariantControl=(inherit)
      settings: CopyFcn=Stateflow.SLINSF.SimulinkMan.removeBlockPreDeleteFcn  PreDeleteFcn=Stateflow.SLINSF.SimulinkMan.unsafePredeleteFcn
  Get Transform : robotmaniplib/Get Transform  RigidBodyTree=franka  SourceBody=hand_link_end  TargetBody=panda_link0  SimulateUsing=Interpreted execution
  Inverse Kinematics{1..5} (5 alike) : robotmaniplib/Inverse Kinematics  RigidBodyTree=franka  EndEffector=hand_link_end  ShowInfo=on  SolverName=BFGS Gradient Projection  EnforceJointLimits=on  MaxIterations=1500  MaxTime=10  GradientTolerance=1e-7  SolutionTolerance=1e-6  StepTolerance=1e-14  ErrorChangeTolerance=1e-12  UseErrorDamping=on  DampingBias=0.0025  SimulateUsing=Interpreted execution
  MATLAB Function : MATLAB Function  TreatAsAtomicUnit=on
  MATLAB Function4 : MATLAB Function  TreatAsAtomicUnit=on
  MATLAB Function6 : MATLAB Function  TreatAsAtomicUnit=on
  Vector Concatenate : Concatenate  NumInputs=5  Mode=Multidimensional array  ConcatenateDimension=2
  panda_pos : Outport
  durTime_panda : Outport  Port=2
  wires:
  panda_state/1 -> MATLAB Function6/1(u), MATLAB Function/5(panda_state)
  tra_pos/1 -> MATLAB Function/1(boxPos)
  tra_ZYX/1 -> MATLAB Function/2(boxZYX)
  sum_actual_pos/1 -> MATLAB Function/3(sumPos)
  sum_actual_ZYX/1 -> MATLAB Function/4(sumZYX)
  state/1 -> MATLAB Function/7(state)
  MATLAB Function/5(durTime) -> durTime_panda/1
  MATLAB Function/4(NWayPoints) -> MATLAB Function4/3(NWayPoint)
  Inverse Kinematics3/1 -> Inverse Kinematics4/3, Vector Concatenate/3
  MATLAB Function6/1(y) -> Get Transform/1
  Vector Concatenate/1 -> panda_pos/1
  MATLAB Function4/1(Pose1) -> Inverse Kinematics1/1
  MATLAB Function4/2(Pose2) -> Inverse Kinematics2/1
  MATLAB Function/3(initialGuess) -> Inverse Kinematics1/3
  MATLAB Function/2(Weights) -> Inverse Kinematics2/2, Inverse Kinematics3/2, Inverse Kinematics5/2, Inverse Kinematics4/2, Inverse Kinematics1/2
  MATLAB Function/1(Pose) -> MATLAB Function4/1(pose_d)
  MATLAB Function4/3(Pose3) -> Inverse Kinematics3/1
  Inverse Kinematics1/1 -> Inverse Kinematics2/3, Vector Concatenate/1
  Inverse Kinematics2/1 -> Inverse Kinematics3/3, Vector Concatenate/2
  Inverse Kinematics4/1 -> Inverse Kinematics5/3, Vector Concatenate/4
  Inverse Kinematics5/1 -> Vector Concatenate/5
  MATLAB Function4/4(Pose4) -> Inverse Kinematics4/1
  MATLAB Function4/5(Pose5) -> Inverse Kinematics5/1
  Get Transform/1 -> MATLAB Function/6(data), MATLAB Function4/2(T)

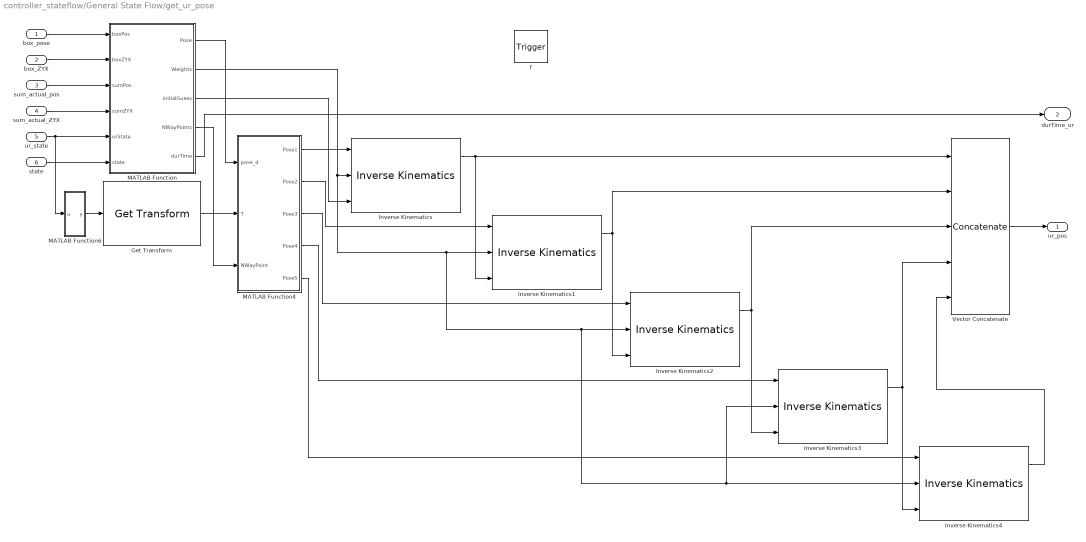
== system controller_stateflow/General State Flow/get_ur_pose ==
  box_pose : Inport  OutDataTypeStr=double  PortDimensions=[3,1]
  box_ZYX : Inport  Port=2  OutDataTypeStr=double  PortDimensions=[3,1]
  sum_actual_pos : Inport  Port=3  OutDataTypeStr=double  PortDimensions=[3,1]
  sum_actual_ZYX : Inport  Port=4  OutDataTypeStr=double  PortDimensions=[3,1]
  ur_state : Inport  Port=5  OutDataTypeStr=double  PortDimensions=[7,1]
  state : Inport  Port=6  OutDataTypeStr=double  PortDimensions=1
  f : TriggerPort  TriggerType=function-call  VariantControl=(inherit)
      settings: CopyFcn=Stateflow.SLINSF.SimulinkMan.removeBlockPreDeleteFcn  PreDeleteFcn=Stateflow.SLINSF.SimulinkMan.unsafePredeleteFcn
  Get Transform : robotmaniplib/Get Transform  RigidBodyTree=ur10e  SourceBody=velvet_link_end  TargetBody=world  SimulateUsing=Interpreted execution
  Inverse Kinematics{,1..4} (5 alike) : robotmaniplib/Inverse Kinematics  RigidBodyTree=ur10e  EndEffector=velvet_link_end  ShowInfo=on  SolverName=BFGS Gradient Projection  EnforceJointLimits=on  MaxIterations=1500  MaxTime=10  GradientTolerance=1e-7  SolutionTolerance=1e-6  StepTolerance=1e-14  ErrorChangeTolerance=1e-12  UseErrorDamping=on  DampingBias=0.0025  SimulateUsing=Interpreted execution
  MATLAB Function : MATLAB Function  TreatAsAtomicUnit=on
  MATLAB Function4 : MATLAB Function  TreatAsAtomicUnit=on
  MATLAB Function6 : MATLAB Function  TreatAsAtomicUnit=on
  Vector Concatenate : Concatenate  NumInputs=5  Mode=Multidimensional array  ConcatenateDimension=2
  ur_pos : Outport
  durTime_ur : Outport  Port=2
  wires:
  ur_state/1 -> MATLAB Function6/1(u), MATLAB Function/5(urState)
  box_pose/1 -> MATLAB Function/1(boxPos)
  box_ZYX/1 -> MATLAB Function/2(boxZYX)
  sum_actual_pos/1 -> MATLAB Function/3(sumPos)
  sum_actual_ZYX/1 -> MATLAB Function/4(sumZYX)
  MATLAB Function/1(Pose) -> MATLAB Function4/1(pose_d)
  MATLAB Function/2(Weights) -> Inverse Kinematics3/2, Inverse Kinematics4/2, Inverse Kinematics2/2, Inverse Kinematics1/2, Inverse Kinematics/2
  MATLAB Function/3(initialGuess) -> Inverse Kinematics/3
  state/1 -> MATLAB Function/6(state)
  Inverse Kinematics/1 -> Inverse Kinematics1/3, Vector Concatenate/1
  Inverse Kinematics1/1 -> Inverse Kinematics2/3, Vector Concatenate/2
  Inverse Kinematics2/1 -> Inverse Kinematics3/3, Vector Concatenate/3
  Inverse Kinematics3/1 -> Inverse Kinematics4/3, Vector Concatenate/4
  Vector Concatenate/1 -> ur_pos/1
  MATLAB Function6/1(y) -> Get Transform/1
  Get Transform/1 -> MATLAB Function4/2(T)
  MATLAB Function/4(NWayPoints) -> MATLAB Function4/3(NWayPoint)
  MATLAB Function4/2(Pose2) -> Inverse Kinematics1/1
  MATLAB Function4/3(Pose3) -> Inverse Kinematics2/1
  MATLAB Function4/4(Pose4) -> Inverse Kinematics3/1
  MATLAB Function4/5(Pose5) -> Inverse Kinematics4/1
  Inverse Kinematics4/1 -> Vector Concatenate/5
  MATLAB Function/5(durTime) -> durTime_ur/1
  MATLAB Function4/1(Pose1) -> Inverse Kinematics/1

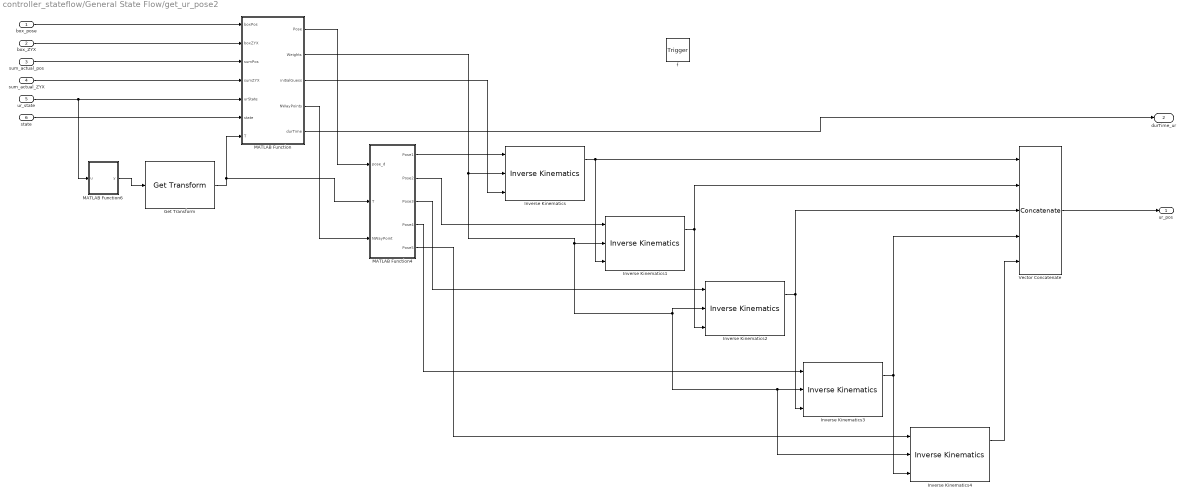
== system controller_stateflow/General State Flow/get_ur_pose2 ==
  box_pose : Inport  OutDataTypeStr=double  PortDimensions=[3,1]
  box_ZYX : Inport  Port=2  OutDataTypeStr=double  PortDimensions=[3,1]
  sum_actual_pos : Inport  Port=3  OutDataTypeStr=double  PortDimensions=[3,1]
  sum_actual_ZYX : Inport  Port=4  OutDataTypeStr=double  PortDimensions=[3,1]
  ur_state : Inport  Port=5  OutDataTypeStr=double  PortDimensions=[7,1]
  state : Inport  Port=6  OutDataTypeStr=double  PortDimensions=1
  f : TriggerPort  TriggerType=function-call  VariantControl=(inherit)
      settings: CopyFcn=Stateflow.SLINSF.SimulinkMan.removeBlockPreDeleteFcn  PreDeleteFcn=Stateflow.SLINSF.SimulinkMan.unsafePredeleteFcn
  Get Transform : robotmaniplib/Get Transform  RigidBodyTree=ur10e  SourceBody=velvet_link_end  TargetBody=world  SimulateUsing=Interpreted execution
  Inverse Kinematics{,1..4} (5 alike) : robotmaniplib/Inverse Kinematics  RigidBodyTree=ur10e  EndEffector=velvet_link_end  ShowInfo=on  SolverName=BFGS Gradient Projection  EnforceJointLimits=on  MaxIterations=1500  MaxTime=10  GradientTolerance=1e-7  SolutionTolerance=1e-6  StepTolerance=1e-14  ErrorChangeTolerance=1e-12  UseErrorDamping=on  DampingBias=0.0025  SimulateUsing=Interpreted execution
  MATLAB Function : MATLAB Function  TreatAsAtomicUnit=on
  MATLAB Function4 : MATLAB Function  TreatAsAtomicUnit=on
  MATLAB Function6 : MATLAB Function  TreatAsAtomicUnit=on
  Vector Concatenate : Concatenate  NumInputs=5  Mode=Multidimensional array  ConcatenateDimension=2
  ur_pos : Outport
  durTime_ur : Outport  Port=2
  wires:
  ur_state/1 -> MATLAB Function/5(urState), MATLAB Function6/1(u)
  box_pose/1 -> MATLAB Function/1(boxPos)
  box_ZYX/1 -> MATLAB Function/2(boxZYX)
  sum_actual_pos/1 -> MATLAB Function/3(sumPos)
  sum_actual_ZYX/1 -> MATLAB Function/4(sumZYX)
  MATLAB Function/1(Pose) -> MATLAB Function4/1(pose_d)
  MATLAB Function/2(Weights) -> Inverse Kinematics4/2, Inverse Kinematics3/2, Inverse Kinematics2/2, Inverse Kinematics1/2, Inverse Kinematics/2
  MATLAB Function/3(initialGuess) -> Inverse Kinematics/3
  state/1 -> MATLAB Function/6(state)
  Inverse Kinematics/1 -> Inverse Kinematics1/3, Vector Concatenate/1
  Inverse Kinematics1/1 -> Inverse Kinematics2/3, Vector Concatenate/2
  Inverse Kinematics2/1 -> Vector Concatenate/3, Inverse Kinematics3/3
  Inverse Kinematics3/1 -> Inverse Kinematics4/3, Vector Concatenate/4
  Vector Concatenate/1 -> ur_pos/1
  MATLAB Function6/1(y) -> Get Transform/1
  Get Transform/1 -> MATLAB Function/7(T), MATLAB Function4/2(T)
  MATLAB Function/4(NWayPoints) -> MATLAB Function4/3(NWayPoint)
  MATLAB Function4/2(Pose2) -> Inverse Kinematics1/1
  MATLAB Function4/3(Pose3) -> Inverse Kinematics2/1
  MATLAB Function4/4(Pose4) -> Inverse Kinematics3/1
  MATLAB Function4/5(Pose5) -> Inverse Kinematics4/1
  Inverse Kinematics4/1 -> Vector Concatenate/5
  MATLAB Function/5(durTime) -> durTime_ur/1
  MATLAB Function4/1(Pose1) -> Inverse Kinematics/1

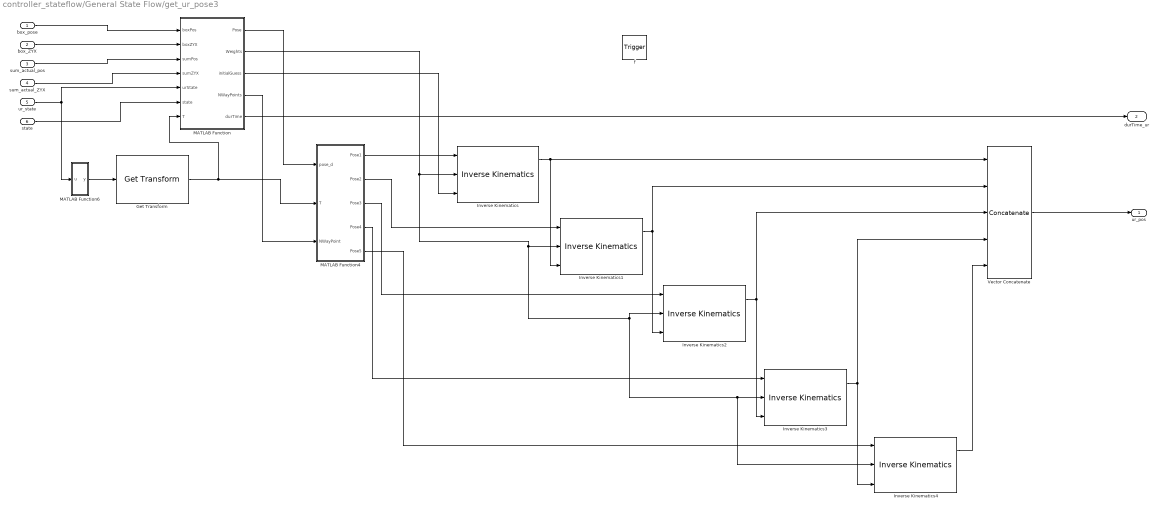
== system controller_stateflow/General State Flow/get_ur_pose3 ==
  box_pose : Inport  OutDataTypeStr=double  PortDimensions=[3,1]
  box_ZYX : Inport  Port=2  OutDataTypeStr=double  PortDimensions=[3,1]
  sum_actual_pos : Inport  Port=3  OutDataTypeStr=double  PortDimensions=[3,1]
  sum_actual_ZYX : Inport  Port=4  OutDataTypeStr=double  PortDimensions=[3,1]
  ur_state : Inport  Port=5  OutDataTypeStr=double  PortDimensions=[7,1]
  state : Inport  Port=6  OutDataTypeStr=double  PortDimensions=1
  f : TriggerPort  TriggerType=function-call  VariantControl=(inherit)
      settings: CopyFcn=Stateflow.SLINSF.SimulinkMan.removeBlockPreDeleteFcn  PreDeleteFcn=Stateflow.SLINSF.SimulinkMan.unsafePredeleteFcn
  Get Transform : robotmaniplib/Get Transform  RigidBodyTree=ur10e  SourceBody=velvet_link_end  TargetBody=world  SimulateUsing=Interpreted execution
  Inverse Kinematics{,1..4} (5 alike) : robotmaniplib/Inverse Kinematics  RigidBodyTree=ur10e  EndEffector=velvet_link_end  ShowInfo=on  SolverName=BFGS Gradient Projection  EnforceJointLimits=on  MaxIterations=1500  MaxTime=10  GradientTolerance=1e-7  SolutionTolerance=1e-6  StepTolerance=1e-14  ErrorChangeTolerance=1e-12  UseErrorDamping=on  DampingBias=0.0025  SimulateUsing=Interpreted execution
  MATLAB Function : MATLAB Function  TreatAsAtomicUnit=on
  MATLAB Function4 : MATLAB Function  TreatAsAtomicUnit=on
  MATLAB Function6 : MATLAB Function  TreatAsAtomicUnit=on
  Vector Concatenate : Concatenate  NumInputs=5  Mode=Multidimensional array  ConcatenateDimension=2
  ur_pos : Outport
  durTime_ur : Outport  Port=2
  wires:
  ur_state/1 -> MATLAB Function/5(urState), MATLAB Function6/1(u)
  box_pose/1 -> MATLAB Function/1(boxPos)
  box_ZYX/1 -> MATLAB Function/2(boxZYX)
  sum_actual_pos/1 -> MATLAB Function/3(sumPos)
  sum_actual_ZYX/1 -> MATLAB Function/4(sumZYX)
  MATLAB Function/1(Pose) -> MATLAB Function4/1(pose_d)
  MATLAB Function/2(Weights) -> Inverse Kinematics4/2, Inverse Kinematics3/2, Inverse Kinematics2/2, Inverse Kinematics1/2, Inverse Kinematics/2
  MATLAB Function/3(initialGuess) -> Inverse Kinematics/3
  state/1 -> MATLAB Function/6(state)
  Inverse Kinematics/1 -> Inverse Kinematics1/3, Vector Concatenate/1
  Inverse Kinematics1/1 -> Inverse Kinematics2/3, Vector Concatenate/2
  Inverse Kinematics2/1 -> Vector Concatenate/3, Inverse Kinematics3/3
  Inverse Kinematics3/1 -> Inverse Kinematics4/3, Vector Concatenate/4
  Vector Concatenate/1 -> ur_pos/1
  MATLAB Function6/1(y) -> Get Transform/1
  Get Transform/1 -> MATLAB Function/7(T), MATLAB Function4/2(T)
  MATLAB Function/4(NWayPoints) -> MATLAB Function4/3(NWayPoint)
  MATLAB Function4/2(Pose2) -> Inverse Kinematics1/1
  MATLAB Function4/3(Pose3) -> Inverse Kinematics2/1
  MATLAB Function4/4(Pose4) -> Inverse Kinematics3/1
  MATLAB Function4/5(Pose5) -> Inverse Kinematics4/1
  Inverse Kinematics4/1 -> Vector Concatenate/5
  MATLAB Function/5(durTime) -> durTime_ur/1
  MATLAB Function4/1(Pose1) -> Inverse Kinematics/1

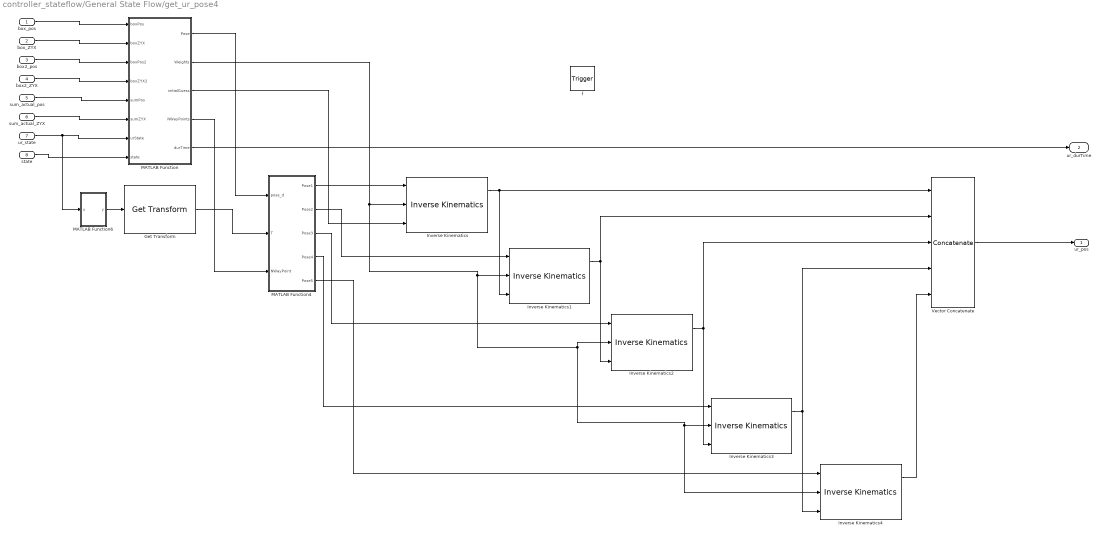
== system controller_stateflow/General State Flow/get_ur_pose4 ==
  box_pos : Inport  OutDataTypeStr=double  PortDimensions=[3,1]
  box_ZYX : Inport  Port=2  OutDataTypeStr=double  PortDimensions=[3,1]
  box2_pos : Inport  Port=3  OutDataTypeStr=double  PortDimensions=[3,1]
  box2_ZYX : Inport  Port=4  OutDataTypeStr=double  PortDimensions=[3,1]
  sum_actual_pos : Inport  Port=5  OutDataTypeStr=double  PortDimensions=[3,1]
  sum_actual_ZYX : Inport  Port=6  OutDataTypeStr=double  PortDimensions=[3,1]
  ur_state : Inport  Port=7  OutDataTypeStr=double  PortDimensions=[7,1]
  state : Inport  Port=8  OutDataTypeStr=double  PortDimensions=1
  f : TriggerPort  TriggerType=function-call  VariantControl=(inherit)
      settings: CopyFcn=Stateflow.SLINSF.SimulinkMan.removeBlockPreDeleteFcn  PreDeleteFcn=Stateflow.SLINSF.SimulinkMan.unsafePredeleteFcn
  Get Transform : robotmaniplib/Get Transform  RigidBodyTree=ur10e  SourceBody=velvet_link_end  TargetBody=world  SimulateUsing=Interpreted execution
  Inverse Kinematics{,1..4} (5 alike) : robotmaniplib/Inverse Kinematics  RigidBodyTree=ur10e  EndEffector=velvet_link_end  ShowInfo=on  SolverName=BFGS Gradient Projection  EnforceJointLimits=on  MaxIterations=1500  MaxTime=10  GradientTolerance=1e-7  SolutionTolerance=1e-6  StepTolerance=1e-14  ErrorChangeTolerance=1e-12  UseErrorDamping=on  DampingBias=0.0025  SimulateUsing=Interpreted execution
  MATLAB Function : MATLAB Function  TreatAsAtomicUnit=on
  MATLAB Function4 : MATLAB Function  TreatAsAtomicUnit=on
  MATLAB Function6 : MATLAB Function  TreatAsAtomicUnit=on
  Vector Concatenate : Concatenate  NumInputs=5  Mode=Multidimensional array  ConcatenateDimension=2
  ur_pos : Outport
  ur_durTime : Outport  Port=2
  wires:
  ur_state/1 -> MATLAB Function6/1(u), MATLAB Function/7(urState)
  box_pos/1 -> MATLAB Function/1(boxPos)
  box_ZYX/1 -> MATLAB Function/2(boxZYX)
  sum_actual_pos/1 -> MATLAB Function/5(sumPos)
  sum_actual_ZYX/1 -> MATLAB Function/6(sumZYX)
  MATLAB Function/1(Pose) -> MATLAB Function4/1(pose_d)
  MATLAB Function/2(Weights) -> Inverse Kinematics4/2, Inverse Kinematics3/2, Inverse Kinematics2/2, Inverse Kinematics1/2, Inverse Kinematics/2
  MATLAB Function/3(initialGuess) -> Inverse Kinematics/3
  Inverse Kinematics/1 -> Inverse Kinematics1/3, Vector Concatenate/1
  Inverse Kinematics1/1 -> Inverse Kinematics2/3, Vector Concatenate/2
  Inverse Kinematics2/1 -> Vector Concatenate/3, Inverse Kinematics3/3
  Inverse Kinematics3/1 -> Inverse Kinematics4/3, Vector Concatenate/4
  Vector Concatenate/1 -> ur_pos/1
  MATLAB Function6/1(y) -> Get Transform/1
  Get Transform/1 -> MATLAB Function4/2(T)
  MATLAB Function/4(NWayPoints) -> MATLAB Function4/3(NWayPoint)
  MATLAB Function4/2(Pose2) -> Inverse Kinematics1/1
  MATLAB Function4/3(Pose3) -> Inverse Kinematics2/1
  MATLAB Function4/4(Pose4) -> Inverse Kinematics3/1
  MATLAB Function4/5(Pose5) -> Inverse Kinematics4/1
  Inverse Kinematics4/1 -> Vector Concatenate/5
  MATLAB Function/5(durTime) -> ur_durTime/1
  MATLAB Function4/1(Pose1) -> Inverse Kinematics/1
  state/1 -> MATLAB Function/8(state)
  box2_pos/1 -> MATLAB Function/3(boxPos2)
  box2_ZYX/1 -> MATLAB Function/4(boxZYX2)

== system controller_stateflow/General State Flow/get_ur_pose_cnvy ==
  tra_pos : Inport  OutDataTypeStr=double  PortDimensions=[3,1]
  tra_ZYX : Inport  Port=2  OutDataTypeStr=double  PortDimensions=[3,1]
  sum_actual_pos : Inport  Port=3  OutDataTypeStr=double  PortDimensions=[3,1]
  sum_actual_ZYX : Inport  Port=4  OutDataTypeStr=double  PortDimensions=[3,1]
  ur_state : Inport  Port=5  OutDataTypeStr=double  PortDimensions=[7,1]
  state : Inport  Port=6  OutDataTypeStr=double  PortDimensions=1
  f : TriggerPort  TriggerType=function-call  VariantControl=(inherit)
      settings: CopyFcn=Stateflow.SLINSF.SimulinkMan.removeBlockPreDeleteFcn  PreDeleteFcn=Stateflow.SLINSF.SimulinkMan.unsafePredeleteFcn
  Get Transform1 : robotmaniplib/Get Transform  RigidBodyTree=ur10e  SourceBody=velvet_link_end  TargetBody=world  SimulateUsing=Interpreted execution
  Inverse Kinematics{,6..9} (5 alike) : robotmaniplib/Inverse Kinematics  RigidBodyTree=ur10e  EndEffector=velvet_link_end  ShowInfo=on  SolverName=BFGS Gradient Projection  EnforceJointLimits=on  MaxIterations=1500  MaxTime=10  GradientTolerance=1e-7  SolutionTolerance=1e-6  StepTolerance=1e-14  ErrorChangeTolerance=1e-12  UseErrorDamping=on  DampingBias=0.0025  SimulateUsing=Interpreted execution
  MATLAB Function1 : MATLAB Function  TreatAsAtomicUnit=on
  MATLAB Function2 : MATLAB Function  TreatAsAtomicUnit=on
  MATLAB Function3 : MATLAB Function  TreatAsAtomicUnit=on
  Vector Concatenate1 : Concatenate  NumInputs=5  Mode=Multidimensional array  ConcatenateDimension=2
  ur_pos : Outport
  durTime_ur : Outport  Port=2
  wires:
  MATLAB Function2/2(Pose2) -> Inverse Kinematics6/1
  MATLAB Function2/4(Pose4) -> Inverse Kinematics8/1
  Inverse Kinematics6/1 -> Inverse Kinematics7/3, Vector Concatenate1/2
  Inverse Kinematics9/1 -> Vector Concatenate1/5
  MATLAB Function3/1(y) -> Get Transform1/1
  MATLAB Function1/3(initialGuess) -> Inverse Kinematics/3
  MATLAB Function2/5(Pose5) -> Inverse Kinematics9/1
  Vector Concatenate1/1 -> ur_pos/1
  MATLAB Function1/2(Weights) -> Inverse Kinematics9/2, Inverse Kinematics8/2, Inverse Kinematics7/2, Inverse Kinematics6/2, Inverse Kinematics/2
  MATLAB Function1/1(Pose) -> MATLAB Function2/1(pose_d)
  MATLAB Function2/1(Pose1) -> Inverse Kinematics/1
  Inverse Kinematics/1 -> Inverse Kinematics6/3, Vector Concatenate1/1
  Inverse Kinematics8/1 -> Inverse Kinematics9/3, Vector Concatenate1/4
  Inverse Kinematics7/1 -> Vector Concatenate1/3, Inverse Kinematics8/3
  MATLAB Function2/3(Pose3) -> Inverse Kinematics7/1
  MATLAB Function1/5(durTime) -> durTime_ur/1
  MATLAB Function1/4(NWayPoints) -> MATLAB Function2/3(NWayPoint)
  Get Transform1/1 -> MATLAB Function2/2(T)
  tra_ZYX/1 -> MATLAB Function1/2(traZYX)
  sum_actual_pos/1 -> MATLAB Function1/3(sumPos)
  sum_actual_ZYX/1 -> MATLAB Function1/4(sumZYX)
  ur_state/1 -> MATLAB Function3/1(u), MATLAB Function1/5(urState)
  state/1 -> MATLAB Function1/6(state)
  tra_pos/1 -> MATLAB Function1/1(traPos)

== system controller_stateflow/Panda Controller Command ==
  time : Inport
  TimeFromStart : Inport  Port=2
  points : Inport  Port=3
  Enable : EnablePort
  Blank Message2 : robotlib/Blank Message  messageClass=Message  entityType=trajectory_msgs/JointTrajectory  messageType=trajectory_msgs/JointTrajectory  SampleTime=inf  legacyBusStruct=off
  Blank Message3 : robotlib/Blank Message  messageClass=Message  entityType=trajectory_msgs/JointTrajectoryPoint  messageType=trajectory_msgs/JointTrajectoryPoint  SampleTime=inf  legacyBusStruct=off
  Publish : robotlib/Publish  topicSource=Select from ROS network  topic=/panda_eff_joint_traj_controller/command  messageType=trajectory_msgs/JointTrajectory  legacyBusStruct=off  messageQueueLength=1
  panda_TrajectoryController_command : MATLAB Function  TreatAsAtomicUnit=on
  wires:
  time/1 -> panda_TrajectoryController_command/1(Time)
  Blank Message3/1 -> panda_TrajectoryController_command/3(msgPoint)
  Blank Message2/1 -> panda_TrajectoryController_command/2(msgIn)
  panda_TrajectoryController_command/1(msgOut) -> Publish/1
  points/1 -> panda_TrajectoryController_command/5(Point_array)
  TimeFromStart/1 -> panda_TrajectoryController_command/4(TimeFromStart)

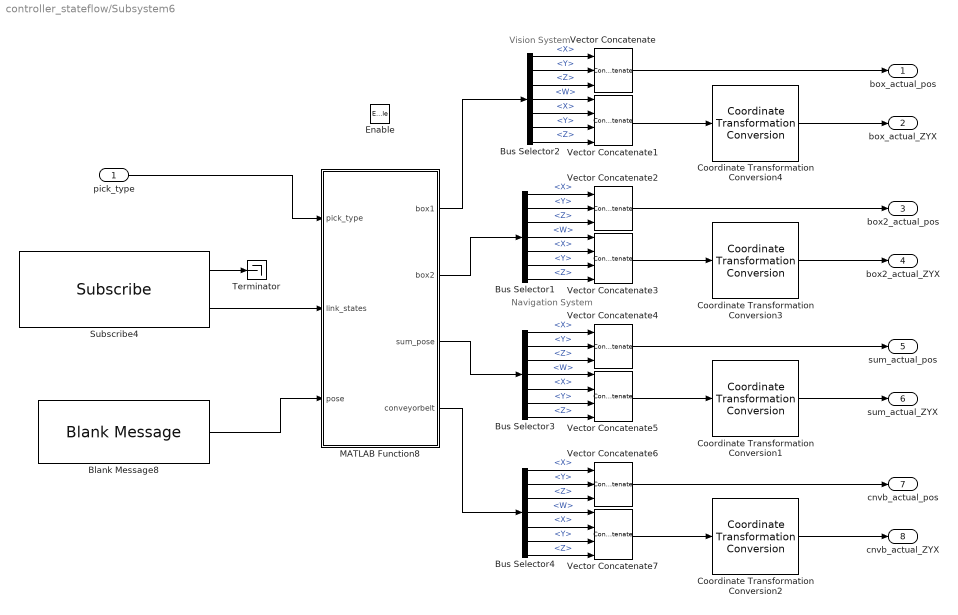
== system controller_stateflow/Subsystem6 ==
  note: Navigation System
  note: Vision System
  pick_type : Inport
  Enable : EnablePort
  Blank Message8 : robotlib/Blank Message  messageClass=Message  entityType=geometry_msgs/Pose  messageType=geometry_msgs/Pose  SampleTime=inf  legacyBusStruct=off
  Bus Selector{1..4} (4 alike) : BusSelector  OutputSignals=Position.X,Position.Y,Position.Z,Orientation.W,Orientation.X,Orientation.Y,Orientation.Z
  Coordinate Transformation Conversion{1..4} (4 alike) : robotcorelib/Coordinate Transformation Conversion  InputRepresentation=Quaternion  InputEulerSequence=ZYX  ShowTrVecInputPort=on  OutputRepresentation=Euler Angles  OutputEulerSequence=ZYX  ShowTrVecOutputPort=on  SimulateUsing=Interpreted execution
      settings: LibrarySourceBlock=roslib/Utilities/Coordinate Transformation Conversion
  MATLAB Function8 : MATLAB Function  TreatAsAtomicUnit=on
  Subscribe4 : robotlib/Subscribe  topicSource=Select from ROS network  topic=/gazebo/link_states  messageType=gazebo_msgs/LinkStates  SampleTime=-1  legacyBusStruct=off  messageQueueLength=1
      settings: LibrarySourceBlock=roslib/ROS/Subscribe
  Terminator : Terminator
  Vector Concatenate{,2,4,6} (4 alike) : Concatenate  NumInputs=3  Mode=Multidimensional array
  Vector Concatenate{1,3,5,7} (4 alike) : Concatenate  NumInputs=4  Mode=Multidimensional array
  box_actual_pos : Outport
  box_actual_ZYX : Outport  Port=2
  box2_actual_pos : Outport  Port=3
  box2_actual_ZYX : Outport  Port=4
  sum_actual_pos : Outport  Port=5
  sum_actual_ZYX : Outport  Port=6
  cnvb_actual_pos : Outport  Port=7
  cnvb_actual_ZYX : Outport  Port=8
  wires:
  Bus Selector2/2 -> Vector Concatenate/2  "<Y>"
  Subscribe4/2 -> MATLAB Function8/2(link_states)
  Vector Concatenate/1 -> box_actual_pos/1
  Coordinate Transformation Conversion2/1 -> cnvb_actual_ZYX/1
  Vector Concatenate6/1 -> cnvb_actual_pos/1
  MATLAB Function8/1(box1) -> Bus Selector2/1
  Coordinate Transformation Conversion4/1 -> box_actual_ZYX/1
  Vector Concatenate7/1 -> Coordinate Transformation Conversion2/1
  Bus Selector3/1 -> Vector Concatenate4/1  "<X>"
  Bus Selector4/1 -> Vector Concatenate6/1  "<X>"
  Blank Message8/1 -> MATLAB Function8/3(pose)
  Vector Concatenate4/1 -> sum_actual_pos/1
  Bus Selector3/3 -> Vector Concatenate4/3  "<Z>"
  Bus Selector4/2 -> Vector Concatenate6/2  "<Y>"
  Coordinate Transformation Conversion1/1 -> sum_actual_ZYX/1
  Vector Concatenate5/1 -> Coordinate Transformation Conversion1/1
  MATLAB Function8/3(sum_pose) -> Bus Selector3/1
  Bus Selector4/3 -> Vector Concatenate6/3  "<Z>"
  Bus Selector2/1 -> Vector Concatenate/1  "<X>"
  Bus Selector3/2 -> Vector Concatenate4/2  "<Y>"
  Vector Concatenate1/1 -> Coordinate Transformation Conversion4/1
  Bus Selector2/3 -> Vector Concatenate/3  "<Z>"
  MATLAB Function8/4(conveyorbelt) -> Bus Selector4/1
  pick_type/1 -> MATLAB Function8/1(pick_type)
  Bus Selector1/3 -> Vector Concatenate2/3  "<Z>"
  Vector Concatenate3/1 -> Coordinate Transformation Conversion3/1
  Bus Selector1/1 -> Vector Concatenate2/1  "<X>"
  Coordinate Transformation Conversion3/1 -> box2_actual_ZYX/1
  MATLAB Function8/2(box2) -> Bus Selector1/1
  Vector Concatenate2/1 -> box2_actual_pos/1
  Bus Selector1/2 -> Vector Concatenate2/2  "<Y>"
  Subscribe4/1 -> Terminator/1
  Bus Selector3/4 -> Vector Concatenate5/1  "<W>"
  Bus Selector3/5 -> Vector Concatenate5/2  "<X>"
  Bus Selector3/6 -> Vector Concatenate5/3  "<Y>"
  Bus Selector3/7 -> Vector Concatenate5/4  "<Z>"
  Bus Selector2/4 -> Vector Concatenate1/1  "<W>"
  Bus Selector2/5 -> Vector Concatenate1/2  "<X>"
  Bus Selector2/6 -> Vector Concatenate1/3  "<Y>"
  Bus Selector2/7 -> Vector Concatenate1/4  "<Z>"
  Bus Selector1/4 -> Vector Concatenate3/1  "<W>"
  Bus Selector1/5 -> Vector Concatenate3/2  "<X>"
  Bus Selector1/6 -> Vector Concatenate3/3  "<Y>"
  Bus Selector1/7 -> Vector Concatenate3/4  "<Z>"
  Bus Selector4/4 -> Vector Concatenate7/1  "<W>"
  Bus Selector4/5 -> Vector Concatenate7/2  "<X>"
  Bus Selector4/6 -> Vector Concatenate7/3  "<Y>"
  Bus Selector4/7 -> Vector Concatenate7/4  "<Z>"
